simulink model "EdLuTSimulink"  (Simulink 8.1)
settings: Solver=ode3  StartTime=0.0  StopTime=1.  FixedStep=0.002  RelTol=1e-3
undefined symbols (not defined in the file or in its folder): frne
undefined symbols (not defined in the file): context, RRedKuKa, RRedKuKadet
libraries: simulink x1
(part 1 of 2)
settings Model: Creator=Sensopac  LastModifiedBy=jgarrido
settings DebuggingCC: StrictBusMsg=Warning
settings SFSimCC: SimParseCustomCode=off

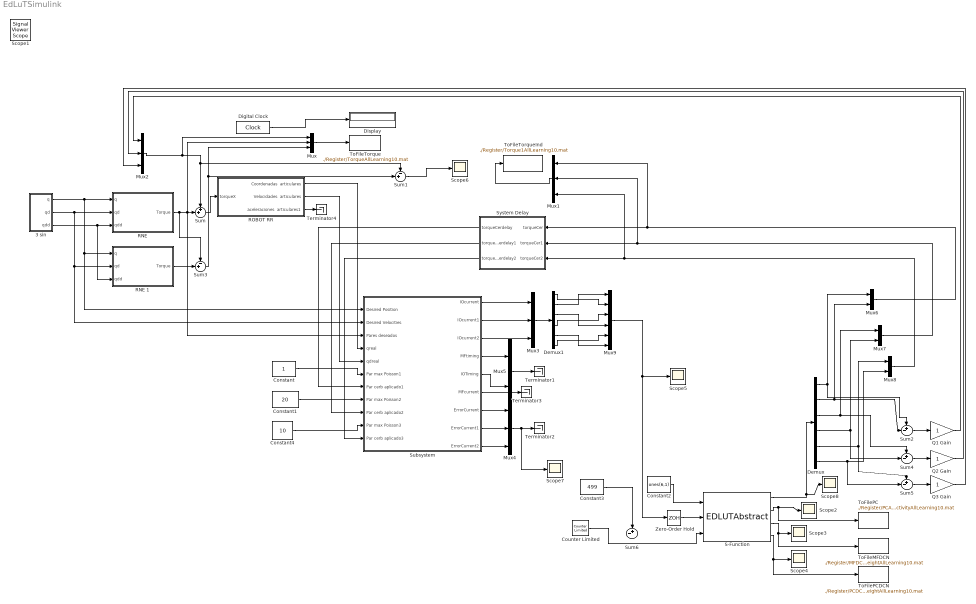
== system EdLuTSimulink ==
  3 sin : Subsystem
  Constant : Constant
  Constant1 : Constant  Value=20
  Constant2 : Constant  Value=ones(6,1)  OutDataTypeStr=double  SampleTime=0.002
  Constant3 : Constant  Value=499  OutDataTypeStr=double  SampleTime=0.002
  Constant4 : Constant  Value=10
  Counter Limited : simulink/Sources/Counter Limited  uplimit=499  tsamp=0.002
  Demux : Demux  Outputs=6
  Demux1 : Demux  Outputs=6
  Digital Clock : DigitalClock  SampleTime=0.002
  Display : Display
  Mux{,1..4} (5 alike) : Mux  Inputs=3
  Mux{5..8} (4 alike) : Mux  Inputs=2
  Mux9 : Mux  Inputs=6
  Q1 Gain : Gain
  Q2 Gain : Gain
  Q3 Gain : Gain
  "RNE " : Subsystem  mask{grav=[ 0 0 9.81], RRed=RRedKuKa}
      mask prompts: grav "Valor de gravedad( 0 0  -9.81)"; RRed "Robot"
      mask help:
      | Este bloque computa la dinamica inversa mediante la utilizacion del algoritmo
      | recursivo Newton Euler (computacionalmente mas eficiente que el metodo de
      | Lagrange-Euler)
      |
      | Se ha de introducir el valor de la gravedad con la que se ha de trabajar (direccion y modulo)
      mask Display:
      | port_label('output',1,'Torque')
      | port_label('input',1,'q')
      | port_label('input',2,'qd')
      | port_label('input',3,'qdd')
      | fprintf('RNE')
  RNE 1 : Subsystem  mask{grav=[ 0 0 9.81], RRed=RRedKuKadet}
      mask prompts: grav "Valor de gravedad( 0 0  -9.81)"; RRed "Robot"
      mask help:
      | Este bloque computa la dinamica inversa mediante la utilizacion del algoritmo
      | recursivo Newton Euler (computacionalmente mas eficiente que el metodo de
      | Lagrange-Euler)
      |
      | Se ha de introducir el valor de la gravedad con la que se ha de trabajar (direccion y modulo)
      mask Display:
      | port_label('output',1,'Torque')
      | port_label('input',1,'q')
      | port_label('input',2,'qd')
      | port_label('input',3,'qdd')
      | fprintf('RNE')
  ROBOT RR : Subsystem  mask{Ciniciales=[0.0  0.1*sin(pi/4)  0.1 0 0 0 0], Viniciales=[2*pi*0.1 2*pi*sin(pi/4)*0.1 0 0 0 0 0], RRed=RRedKuKadet}
      mask prompts: Ciniciales "Condiciones iniciales q"; Viniciales "Velocidades iniciales qd"; RRed "Robot"
      mask help: Modelado del brazo robotico mediante dinamica rigida
  S-Function : S-Function  FunctionName=EDLUTAbstract  Parameters=ParamFile NumberOfJoints NumberOfStates WeightFile WeightInitFile  EnableBusSupport=off  mask{ParamFile='Parametros.txt', NumberOfJoints=6, NumberOfStates=500, WeightFile='./Register/WeightsOnlyPC2_5.dat', WeightInitFile='./InitialWeights25.dat'}
      mask prompts: ParamFile "Learning Configuration File"; NumberOfJoints "Number Of Joints"; NumberOfStates "Number Of States"; WeightFile "Final Weight File"; WeightInitFile "Initial Weight File"
      mask Display:
      | port_label('input',1,'MFAct')
      | port_label('input',2,'Error')
      | port_label('input',3,'State')
      | port_label('output',1,'DCNAct')
      | port_label('output',2,'PCAct')
      | port_label('output',3,'MFWeight')
      | port_label('output',4,'PCWeight')
  Scope{2..8} (7 alike) : Scope
      Scope2 settings: TimeRange=10  YMin=0.3  YMax=1  SaveName=ScopeData3
      Scope3 settings: TimeRange=10  YMin=0  YMax=0.65  SaveName=ScopeData4
      Scope4 settings: TimeRange=20  YMin=6  YMax=80  SaveName=ScopeData5
      Scope5 settings: TimeRange=10  YMin=0  YMax=1
      Scope6 settings: TimeRange=20  YMin=-20  YMax=22.5  SaveName=ScopeData6
      Scope7 settings: TimeRange=10  YMin=-3  YMax=4  SaveName=ScopeData8
      Scope8 settings: TimeRange=10  YMin=0  YMax=17  SaveName=ScopeData9
  Subsystem : Subsystem
  Sum : Sum  Inputs=++|
  Sum1 : Sum  Inputs=-+|
  Sum2 : Sum  Inputs=+-|
  Sum3 : Sum  Inputs=-+|
  Sum4 : Sum  Inputs=+-|
  Sum5 : Sum  Inputs=+-|
  Sum6 : Sum  Inputs=+-|  OutDataTypeStr=uint16
  System Delay : Subsystem  mask{delta1=0}
      mask prompts: delta1 "Delay delta1"
  Terminator{1..4} (4 alike) : Terminator
  ToFileMFDCN : ToFile  Filename=./Register/MFDCNWeightAllLearning10.mat
  ToFilePC : ToFile  Filename=./Register/PCActivityAllLearning10.mat
  ToFilePCDCN : ToFile  Filename=./Register/PCDCNWeightAllLearning10.mat
  ToFileTorque : ToFile  Filename=./Register/TorqueAllLearning10.mat
  ToFileTorqueInd : ToFile  Filename=./Register/Torque1AllLearning10.mat
  Zero-Order Hold : ZeroOrderHold  SampleTime=0.002
  Scope1 : SignalViewerScope  IOType=viewer  RefreshTime=0.035000
  wires:
  3 sin/1(q) -> "RNE "/1(q), Subsystem/1(Desired Position), RNE 1/1(q)
  3 sin/2(qd) -> "RNE "/2(qd), Subsystem/2(Desired Velocities), RNE 1/2(qd)
  3 sin/3(qdd) -> "RNE "/3(qdd), RNE 1/3(qdd)
  "RNE "/1(Torque) -> Sum3/1, Sum/2, Mux/2, Subsystem/3(Pares deseados)
  ROBOT RR/1(Coordenadas  articulares) -> Subsystem/4(qreal)
  ROBOT RR/2(Velocidades  articulares) -> Subsystem/5(qdreal)
  Constant/1 -> Subsystem/6(Par max Poisson1)
  Constant1/1 -> Subsystem/8(Par max Poisson2)
  Constant4/1 -> Subsystem/10(Par max Poisson3)
  System Delay/1(torqueCerdelay) -> Subsystem/7(Par cerb aplicado1)
  System Delay/2(torqueCerdelay1) -> Subsystem/9(Par cerb aplicado2)
  System Delay/3(torqueCerdelay2) -> Subsystem/11(Par cerb aplicado3)
  Sum/1 -> ROBOT RR/1(torqueX)
  Subsystem/6(MFcurrent) -> Terminator3/1
  ROBOT RR/3(aceleraciones  articulares1) -> Terminator4/1
  Mux2/1 -> Sum/1, Sum1/1, Mux/1
  Mux/1 -> ToFileTorque/1
  Mux1/1 -> ToFileTorqueInd/1
  Constant2/1 -> S-Function/1
  S-Function/1 -> Demux/1, Scope8/1
  S-Function/2 -> Scope2/1, ToFilePC/1
  S-Function/3 -> Scope3/1, ToFileMFDCN/1
  S-Function/4 -> Scope4/1, ToFilePCDCN/1
  RNE 1/1(Torque) -> Sum3/2
  Sum3/1 -> Sum1/2, Mux/3
  Zero-Order Hold/1 -> S-Function/2
  Mux6/1 -> System Delay/1(torqueCer), Mux1/1
  Mux7/1 -> System Delay/2(torqueCer1), Mux1/2
  Mux8/1 -> System Delay/3(torqueCer2), Mux1/3
  Sum1/1 -> Scope6/1
  Demux/1 -> Sum2/1, Mux6/1
  Demux/3 -> Sum4/1, Mux7/1
  Demux/5 -> Sum5/1, Mux8/1
  Demux/6 -> Sum5/2, Mux8/2
  Demux/4 -> Sum4/2, Mux7/2
  Demux/2 -> Sum2/2, Mux6/2
  Mux5/1 -> Terminator1/1
  Mux4/1 -> Terminator2/1, Scope7/1
  Subsystem/5(IOTiming) -> Mux5/2
  Subsystem/4(MFtiming) -> Mux5/1
  Subsystem/7(ErrorCurrent) -> Mux4/1
  Subsystem/8(ErrorCurrent1) -> Mux4/2
  Subsystem/9(ErrorCurrent2) -> Mux4/3
  Mux3/1 -> Demux1/1
  Mux9/1 -> Zero-Order Hold/1, Scope5/1
  Demux1/2 -> Mux9/1
  Demux1/1 -> Mux9/2
  Demux1/3 -> Mux9/4
  Demux1/4 -> Mux9/3
  Demux1/5 -> Mux9/6
  Demux1/6 -> Mux9/5
  Subsystem/1(IOcurrent) -> Mux3/1
  Subsystem/2(IOcurrent1) -> Mux3/2
  Subsystem/3(IOcurrent2) -> Mux3/3
  Digital Clock/1 -> Display/1
  Constant3/1 -> Sum6/1
  Counter Limited/1 -> S-Function/3
  Sum2/1 -> Q1 Gain/1
  Q1 Gain/1 -> Mux2/1
  Sum4/1 -> Q2 Gain/1
  Q2 Gain/1 -> Mux2/2
  Sum5/1 -> Q3 Gain/1
  Q3 Gain/1 -> Mux2/3

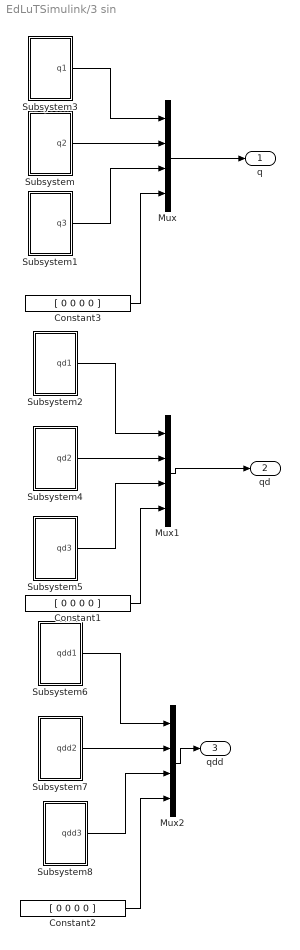
== system EdLuTSimulink/3 sin ==
  Constant1 : Constant  Value=[ 0 0 0 0 ]
  Constant2 : Constant  Value=[ 0 0 0 0 ]
  Constant3 : Constant  Value=[ 0 0 0 0 ]
  Mux : Mux
  Mux1 : Mux
  Mux2 : Mux
  Subsystem : Subsystem
  Subsystem1 : Subsystem
  Subsystem2 : Subsystem
  Subsystem3 : Subsystem
  Subsystem4 : Subsystem
  Subsystem5 : Subsystem
  Subsystem6 : Subsystem
  Subsystem7 : Subsystem
  Subsystem8 : Subsystem
  q : Outport
  qd : Outport  Port=2
  qdd : Outport  Port=3
  wires:
  Mux2/1 -> qdd/1
  Mux1/1 -> qd/1
  Mux/1 -> q/1
  Subsystem3/1(q1) -> Mux/1
  Subsystem/1(q2) -> Mux/2
  Subsystem1/1(q3) -> Mux/3
  Subsystem2/1(qd1) -> Mux1/1
  Subsystem4/1(qd2) -> Mux1/2
  Subsystem5/1(qd3) -> Mux1/3
  Subsystem6/1(qdd1) -> Mux2/1
  Subsystem7/1(qdd2) -> Mux2/2
  Subsystem8/1(qdd3) -> Mux2/3
  Constant3/1 -> Mux/4
  Constant1/1 -> Mux1/4
  Constant2/1 -> Mux2/4

== system EdLuTSimulink/RNE  ==
  q : Inport
  qd : Inport  Port=2
  qdd : Inport  Port=3
  Mux : Mux  Inputs=3
  S-Function : S-Function  FunctionName=Select  Parameters=RRed  EnableBusSupport=off
  S-Function1 : S-Function  FunctionName=Select  Parameters=RRed  EnableBusSupport=off
  S-Function2 : S-Function  FunctionName=Select  Parameters=RRed  EnableBusSupport=off
  rne : MATLABFcn  MATLABFcn=frne(RRed, u(1:RRed.n)', u(RRed.n+1:2*RRed.n)', u(2* RRed.n+1:3*RRed.n)',grav)  OutputDimensions=RRed.n
  Torque : Outport
  wires:
  qdd/1 -> S-Function2/1
  rne/1 -> Torque/1
  q/1 -> S-Function/1
  Mux/1 -> rne/1
  qd/1 -> S-Function1/1
  S-Function/1 -> Mux/1
  S-Function1/1 -> Mux/2
  S-Function2/1 -> Mux/3

== system EdLuTSimulink/RNE 1 ==
  q : Inport
  qd : Inport  Port=2
  qdd : Inport  Port=3
  Mux : Mux  Inputs=3
  S-Function : S-Function  FunctionName=Select  Parameters=RRed  EnableBusSupport=off
  S-Function1 : S-Function  FunctionName=Select  Parameters=RRed  EnableBusSupport=off
  S-Function2 : S-Function  FunctionName=Select  Parameters=RRed  EnableBusSupport=off
  rne : MATLABFcn  MATLABFcn=frne(RRed, u(1:RRed.n)', u(RRed.n+1:2*RRed.n)', u(2* RRed.n+1:3*RRed.n)',grav)  OutputDimensions=RRed.n
  Torque : Outport
  wires:
  qdd/1 -> S-Function2/1
  rne/1 -> Torque/1
  q/1 -> S-Function/1
  Mux/1 -> rne/1
  qd/1 -> S-Function1/1
  S-Function/1 -> Mux/1
  S-Function1/1 -> Mux/2
  S-Function2/1 -> Mux/3

== system EdLuTSimulink/ROBOT RR ==
  torqueX : Inport
  Constant : Constant  Value=Ciniciales
  Constant1 : Constant  Value=Viniciales
  Integrator : Integrator  ExternalReset=falling  InitialConditionSource=external
  Integrator1 : Integrator  ExternalReset=falling  InitialConditionSource=external
  Mux : Mux  Inputs=3
  Reset Contidions : Subsystem  mask{T=1}
      mask prompts: T "Period"
      mask Display: port_label ('output',1,'FallingReset')
  S-Function : S-Function  FunctionName=CINDIR  Parameters=RRed  EnableBusSupport=off
  S-Function1 : S-Function  FunctionName=Select  Parameters=RRed  EnableBusSupport=off
  S-Function2 : S-Function  FunctionName=Select  Parameters=RRed  EnableBusSupport=off
  Coordenadas  articulares : Outport
  Velocidades  articulares : Outport  Port=2
  aceleraciones  articulares1 : Outport  Port=3
  wires:
  torqueX/1 -> Mux/3
  Integrator/1 -> Integrator1/1, Mux/2, Velocidades  articulares/1  "qd"
  Mux/1 -> S-Function/1
  S-Function/1 -> Integrator/1, aceleraciones  articulares1/1  "qdd"
  Constant/1 -> S-Function1/1
  Integrator1/1 -> Mux/1, Coordenadas  articulares/1  "q"
  S-Function1/1 -> Integrator1/3
  S-Function2/1 -> Integrator/3
  Constant1/1 -> S-Function2/1
  Reset Contidions/1(Out1) -> Integrator1/2, Integrator/2

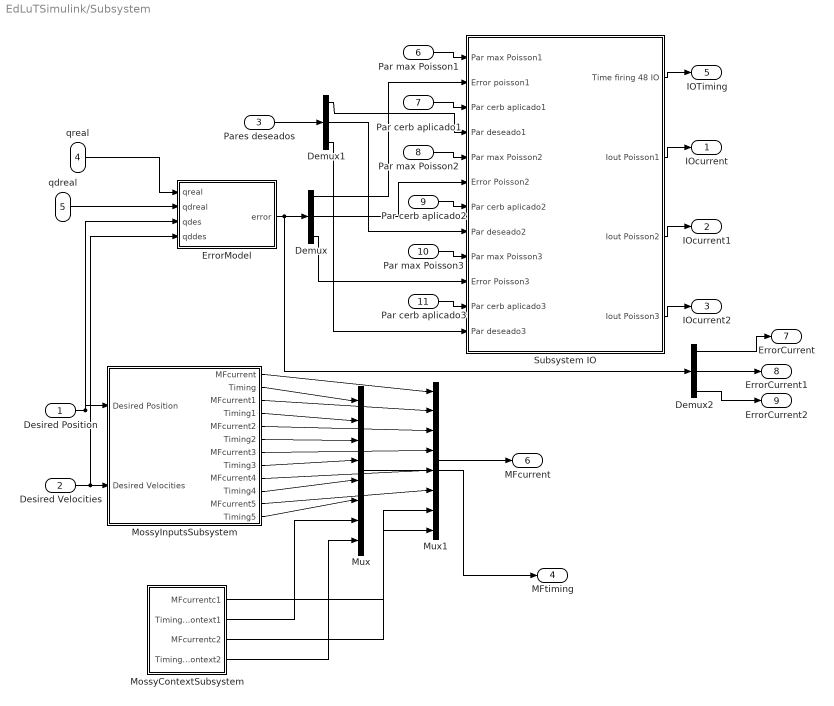
== system EdLuTSimulink/Subsystem ==
  Desired Position : Inport
  Desired Velocities : Inport  Port=2
  Pares deseados : Inport  Port=3
  qreal : Inport  Port=4
  qdreal : Inport  Port=5
  Par max Poisson1 : Inport  Port=6
  Par cerb aplicado1 : Inport  Port=7
  Par max Poisson2 : Inport  Port=8
  Par cerb aplicado2 : Inport  Port=9
  Par max Poisson3 : Inport  Port=10
  Par cerb aplicado3 : Inport  Port=11
  Demux : Demux  Outputs=3
  Demux1 : Demux  Outputs=3
  Demux2 : Demux  Outputs=3
  ErrorModel : Subsystem
  MossyContextSubsystem : Subsystem
  MossyInputsSubsystem : Subsystem
  Mux : Mux  Inputs=8
  Mux1 : Mux  Inputs=8
  Subsystem IO : Subsystem
  IOcurrent : Outport
  IOcurrent1 : Outport  Port=2
  IOcurrent2 : Outport  Port=3
  MFtiming : Outport  Port=4
  IOTiming : Outport  Port=5
  MFcurrent : Outport  Port=6
  ErrorCurrent : Outport  Port=7
  ErrorCurrent1 : Outport  Port=8
  ErrorCurrent2 : Outport  Port=9
  wires:
  Desired Position/1 -> MossyInputsSubsystem/1(Desired Position), ErrorModel/3(qdes)
  Desired Velocities/1 -> MossyInputsSubsystem/2(Desired Velocities), ErrorModel/4(qddes)
  Par max Poisson1/1 -> Subsystem IO/1(Par max Poisson1)
  Subsystem IO/1(Time firing 48 IO) -> IOTiming/1
  Demux/1 -> Subsystem IO/2(Error poisson1)
  Par cerb aplicado1/1 -> Subsystem IO/3(Par cerb aplicado1)
  Demux1/1 -> Subsystem IO/4(Par deseado1)
  Subsystem IO/2(Iout Poisson1) -> IOcurrent/1
  Par max Poisson2/1 -> Subsystem IO/5(Par max Poisson2)
  Demux/2 -> Subsystem IO/6(Error Poisson2)
  Par cerb aplicado2/1 -> Subsystem IO/7(Par cerb aplicado2)
  Subsystem IO/3(Iout Poisson2) -> IOcurrent1/1
  Par max Poisson3/1 -> Subsystem IO/9(Par max Poisson3)
  Demux/3 -> Subsystem IO/10(Error Poisson3)
  Par cerb aplicado3/1 -> Subsystem IO/11(Par cerb aplicado3)
  Subsystem IO/4(Iout Poisson3) -> IOcurrent2/1
  Demux1/3 -> Subsystem IO/12(Par deseado3)
  Pares deseados/1 -> Demux1/1
  ErrorModel/1(error) -> Demux/1, Demux2/1
  qreal/1 -> ErrorModel/1(qreal)
  qdreal/1 -> ErrorModel/2(qdreal)
  Demux1/2 -> Subsystem IO/8(Par deseado2)
  MossyInputsSubsystem/2(Timing) -> Mux/1
  MossyInputsSubsystem/4(Timing1) -> Mux/2
  MossyInputsSubsystem/6(Timing2) -> Mux/3
  MossyInputsSubsystem/8(Timing3) -> Mux/4
  MossyInputsSubsystem/10(Timing4) -> Mux/5
  MossyInputsSubsystem/12(Timing5) -> Mux/6
  MossyContextSubsystem/2(TimingContext1) -> Mux/7
  MossyContextSubsystem/4(TimingContext2) -> Mux/8
  Mux/1 -> MFtiming/1
  MossyInputsSubsystem/1(MFcurrent) -> Mux1/1
  MossyInputsSubsystem/3(MFcurrent1) -> Mux1/2
  MossyInputsSubsystem/5(MFcurrent2) -> Mux1/3
  MossyInputsSubsystem/7(MFcurrent3) -> Mux1/4
  MossyInputsSubsystem/9(MFcurrent4) -> Mux1/5
  MossyInputsSubsystem/11(MFcurrent5) -> Mux1/6
  MossyContextSubsystem/1(MFcurrentc1) -> Mux1/7
  MossyContextSubsystem/3(MFcurrentc2) -> Mux1/8
  Mux1/1 -> MFcurrent/1
  Demux2/1 -> ErrorCurrent/1
  Demux2/2 -> ErrorCurrent1/1
  Demux2/3 -> ErrorCurrent2/1

== system EdLuTSimulink/System Delay ==
  torqueCer : Inport
  torqueCer1 : Inport  Port=2
  torqueCer2 : Inport  Port=3
  Transport Delay1 : TransportDelay  DelayTime=delta1
  Transport Delay2 : TransportDelay  DelayTime=delta1
  Transport Delay3 : TransportDelay  DelayTime=delta1
  torqueCerdelay : Outport
  torqueCerdelay1 : Outport  Port=2
  torqueCerdelay2 : Outport  Port=3
  wires:
  torqueCer/1 -> Transport Delay1/1
  Transport Delay1/1 -> torqueCerdelay/1
  torqueCer1/1 -> Transport Delay2/1
  Transport Delay2/1 -> torqueCerdelay1/1
  torqueCer2/1 -> Transport Delay3/1
  Transport Delay3/1 -> torqueCerdelay2/1

== system EdLuTSimulink/3 sin/Subsystem ==
  Constant1 : Constant  Value=0.1
  Constant2 : Constant  Value=pi/4
  Constant3 : Constant  Value=2*pi
  Digital Clock : DigitalClock  SampleTime=0.002
  Product : Product  RndMeth=Zero
  Product2 : Product  RndMeth=Zero
  Sum : Sum  Inputs=|++
  Trigonometric Function : Trigonometry
  q2 : Outport
  wires:
  Sum/1 -> Trigonometric Function/1
  Constant2/1 -> Sum/1
  Product2/1 -> Sum/2
  Product/1 -> q2/1
  Trigonometric Function/1 -> Product/2
  Constant3/1 -> Product2/1
  Digital Clock/1 -> Product2/2
  Constant1/1 -> Product/1

== system EdLuTSimulink/3 sin/Subsystem1 ==
  Constant2 : Constant  Value=0.1
  Constant3 : Constant  Value=pi/2
  Constant4 : Constant  Value=2*pi
  Digital Clock : DigitalClock  SampleTime=0.002
  Product : Product  RndMeth=Zero
  Product2 : Product  RndMeth=Zero
  Sum : Sum  Inputs=|++
  Trigonometric Function : Trigonometry
  q3 : Outport
  wires:
  Sum/1 -> Trigonometric Function/1
  Constant3/1 -> Sum/1
  Product2/1 -> Sum/2
  Product/1 -> q3/1
  Trigonometric Function/1 -> Product/2
  Constant4/1 -> Product2/1
  Digital Clock/1 -> Product2/2
  Constant2/1 -> Product/1

== system EdLuTSimulink/3 sin/Subsystem2 ==
  Constant1 : Constant  Value=0.1*2*pi
  Constant3 : Constant  Value=2*pi
  Digital Clock : DigitalClock  SampleTime=0.002
  Product : Product  RndMeth=Zero
  Product2 : Product  RndMeth=Zero
  Trigonometric Function : Trigonometry  Operator=cos
  qd1 : Outport
  wires:
  Product/1 -> qd1/1
  Trigonometric Function/1 -> Product/2
  Constant3/1 -> Product2/1
  Product2/1 -> Trigonometric Function/1
  Digital Clock/1 -> Product2/2
  Constant1/1 -> Product/1

== system EdLuTSimulink/3 sin/Subsystem3 ==
  Constant1 : Constant  Value=0.1
  Constant3 : Constant  Value=2*pi
  Digital Clock : DigitalClock  SampleTime=0.002
  Product : Product  RndMeth=Zero
  Product2 : Product  RndMeth=Zero
  Trigonometric Function : Trigonometry
  q1 : Outport
  wires:
  Product/1 -> q1/1
  Trigonometric Function/1 -> Product/2
  Constant3/1 -> Product2/1
  Product2/1 -> Trigonometric Function/1
  Digital Clock/1 -> Product2/2
  Constant1/1 -> Product/1

== system EdLuTSimulink/3 sin/Subsystem4 ==
  Constant1 : Constant  Value=0.1*2*pi
  Constant2 : Constant  Value=pi/4
  Constant3 : Constant  Value=2*pi
  Digital Clock : DigitalClock  SampleTime=0.002
  Product : Product  RndMeth=Zero
  Product2 : Product  RndMeth=Zero
  Sum : Sum  Inputs=|++
  Trigonometric Function : Trigonometry  Operator=cos
  qd2 : Outport
  wires:
  Sum/1 -> Trigonometric Function/1
  Constant2/1 -> Sum/1
  Product2/1 -> Sum/2
  Product/1 -> qd2/1
  Trigonometric Function/1 -> Product/2
  Constant3/1 -> Product2/1
  Digital Clock/1 -> Product2/2
  Constant1/1 -> Product/1

== system EdLuTSimulink/3 sin/Subsystem5 ==
  Constant1 : Constant  Value=0.1*2*pi
  Constant3 : Constant  Value=pi/2
  Constant4 : Constant  Value=2*pi
  Digital Clock : DigitalClock  SampleTime=0.002
  Product : Product  RndMeth=Zero
  Product2 : Product  RndMeth=Zero
  Sum : Sum  Inputs=|++
  Trigonometric Function : Trigonometry  Operator=cos
  qd3 : Outport
  wires:
  Sum/1 -> Trigonometric Function/1
  Constant3/1 -> Sum/1
  Product2/1 -> Sum/2
  Product/1 -> qd3/1
  Trigonometric Function/1 -> Product/2
  Constant4/1 -> Product2/1
  Digital Clock/1 -> Product2/2
  Constant1/1 -> Product/1

== system EdLuTSimulink/3 sin/Subsystem6 ==
  Constant1 : Constant  Value=-0.1*4*pi^2
  Constant3 : Constant  Value=2*pi
  Digital Clock : DigitalClock  SampleTime=0.002
  Product : Product  RndMeth=Zero
  Product2 : Product  RndMeth=Zero
  Trigonometric Function : Trigonometry
  qdd1 : Outport
  wires:
  Product/1 -> qdd1/1
  Trigonometric Function/1 -> Product/2
  Constant3/1 -> Product2/1
  Product2/1 -> Trigonometric Function/1
  Digital Clock/1 -> Product2/2
  Constant1/1 -> Product/1

== system EdLuTSimulink/3 sin/Subsystem7 ==
  Constant1 : Constant  Value=-0.1*4*pi^2
  Constant2 : Constant  Value=pi/4
  Constant3 : Constant  Value=2*pi
  Digital Clock : DigitalClock  SampleTime=0.002
  Product : Product  RndMeth=Zero
  Product2 : Product  RndMeth=Zero
  Sum : Sum  Inputs=|++
  Trigonometric Function : Trigonometry
  qdd2 : Outport
  wires:
  Sum/1 -> Trigonometric Function/1
  Constant2/1 -> Sum/1
  Product2/1 -> Sum/2
  Product/1 -> qdd2/1
  Trigonometric Function/1 -> Product/2
  Constant3/1 -> Product2/1
  Digital Clock/1 -> Product2/2
  Constant1/1 -> Product/1

== system EdLuTSimulink/3 sin/Subsystem8 ==
  Constant1 : Constant  Value=-0.1*4*pi^2
  Constant3 : Constant  Value=pi/2
  Constant4 : Constant  Value=2*pi
  Digital Clock : DigitalClock  SampleTime=0.002
  Product : Product  RndMeth=Zero
  Product2 : Product  RndMeth=Zero
  Sum : Sum  Inputs=|++
  Trigonometric Function : Trigonometry
  qdd3 : Outport
  wires:
  Sum/1 -> Trigonometric Function/1
  Constant3/1 -> Sum/1
  Product2/1 -> Sum/2
  Product/1 -> qdd3/1
  Trigonometric Function/1 -> Product/2
  Constant4/1 -> Product2/1
  Digital Clock/1 -> Product2/2
  Constant1/1 -> Product/1

== system EdLuTSimulink/ROBOT RR/Reset Contidions ==
  Constant2 : Constant  Value=T
  Digital Clock : DigitalClock  SampleTime=0.002
  Math Function : Math  Operator=mod  OutputSignalType=real  SaturateOnIntegerOverflow=on
  Out1 : Outport
  wires:
  Digital Clock/1 -> Math Function/1
  Constant2/1 -> Math Function/2
  Math Function/1 -> Out1/1

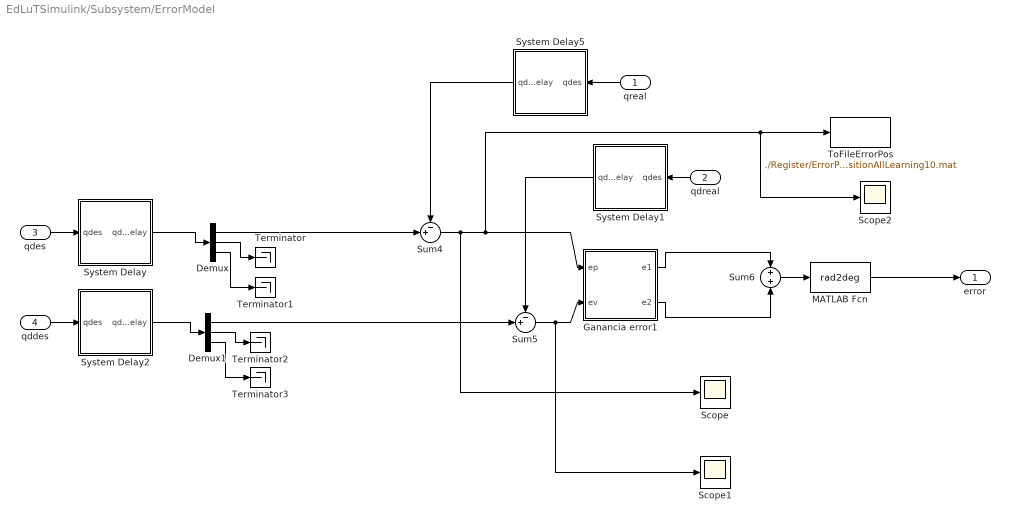
== system EdLuTSimulink/Subsystem/ErrorModel ==
  qreal : Inport
  qdreal : Inport  Port=2
  qdes : Inport  Port=3
  qddes : Inport  Port=4
  Demux : Demux  Outputs=3
  Demux1 : Demux  Outputs=3
  Ganancia error1 : Subsystem  mask{KP1=1, KP2=12, KP3=6, KV1=2, KV2=10, KV3=5}
      mask prompts: KP1 "Constante error de posición1"; KP2 "Constante error de posición2"; KP3 "Constante error de posición3"; KV1 "Constante error de velocidad1"; KV2 "Constante error de velocidad2"; KV3 "Constante error de velocidad3"
  MATLAB Fcn : MATLABFcn  MATLABFcn=rad2deg
  Scope : Scope
      settings: YMin=-0.02  YMax=0.15
  Scope1 : Scope
      settings: TimeRange=20  YMin=-0.05  YMax=0.375  SaveName=ScopeData2
  Scope2 : Scope
      settings: TimeRange=20  YMin=-0.005  YMax=0.0425  SaveName=ScopeData7
  Sum4 : Sum  Inputs=-+|
  Sum5 : Sum  Inputs=-+|
  Sum6 : Sum
  System Delay : Subsystem  mask{delta1=0, delta2=0, qinicial=[0.0  0.1*sin(pi/4)  0.1 0 0 0 0]}
      mask prompts: delta1 "Primer delay delta1"; delta2 "Segundo delay delta2"; qinicial "Posición inicial [q1 q2 q3 q4 q5 q6 q7]"
  System Delay1 : Subsystem  mask{delta1=0, delta2=0, qinicial=[2*pi*0.1 2*pi*sin(pi/4)*0.1 0]}
      mask prompts: delta1 "Primer delay delta1"; delta2 "Segundo delay delta2"; qinicial "Velocidad inicial [qd1 qd2 qd3]"
  System Delay2 : Subsystem  mask{delta1=0, delta2=0, qinicial=[2*pi*0.1 2*pi*sin(pi/4)*0.1 0 0 0 0 0]}
      mask prompts: delta1 "Primer delay delta1"; delta2 "Segundo delay delta2"; qinicial "Velocidad inicial [qd1 qd2 qd3 qd4 qd5 qd6 qd7]"
  System Delay5 : Subsystem  mask{delta1=0, delta2=0, qinicial=[0.0  0.1*sin(pi/4)  0.1]}
      mask prompts: delta1 "Primer delay delta1"; delta2 "Segundo delay delta2"; qinicial "Posición inicial [q1 q2 q3 ]"
  Terminator{,1..3} (4 alike) : Terminator
  ToFileErrorPos : ToFile  Filename=./Register/ErrorPositionAllLearning10.mat
  error : Outport
  wires:
  Sum4/1 -> Ganancia error1/1(ep), Scope2/1, ToFileErrorPos/1, Scope/1
  Sum5/1 -> Ganancia error1/2(ev), Scope1/1
  Ganancia error1/1(e1) -> Sum6/1
  Ganancia error1/2(e2) -> Sum6/2
  qreal/1 -> System Delay5/1(qdes)
  qdreal/1 -> System Delay1/1(qdes)
  qdes/1 -> System Delay/1(qdes)
  qddes/1 -> System Delay2/1(qdes)
  Sum6/1 -> MATLAB Fcn/1
  System Delay5/1(qdesdelay) -> Sum4/1
  System Delay1/1(qdesdelay) -> Sum5/1
  System Delay/1(qdesdelay) -> Demux/1
  System Delay2/1(qdesdelay) -> Demux1/1
  Demux/1 -> Sum4/2
  Demux1/1 -> Sum5/2
  Demux/2 -> Terminator/1
  Demux/3 -> Terminator1/1
  Demux1/2 -> Terminator2/1
  Demux1/3 -> Terminator3/1
  MATLAB Fcn/1 -> error/1

== system EdLuTSimulink/Subsystem/MossyContextSubsystem ==
  Contexto : Subsystem  mask{Variable_Contexto=context, Variable_Contexto1=context}
      mask prompts: Variable_Contexto "Variable de  contexto 1"; Variable_Contexto1 "Variable de contexto 2"
  Demux : Demux  Outputs=2
  Mossy1 : Subsystem  mask{R=5, Taum=0.02, Um0=0, Uth=1, Ureset=0, Trefrac=0, NumMFs=4}
      mask prompts: R "Valor R"; Um0 "Valor inicial de Um"; Uth "Tensión Th"; Ureset "Tensión Reset"; Trefrac "Tiempo Refractario"; NumMFs "Numero de MFs"
      mask Display:
      | port_label('input',1,'MFs inputs')
      | port_label('output',1,'MFs potential')
      | port_label('output',2,'Firing MFs')
  Mossy7 : Subsystem  mask{R=5, Taum=0.02, Um0=0, Uth=1, Ureset=0, Trefrac=0, NumMFs=4}
      mask prompts: R "Valor R"; Um0 "Valor inicial de Um"; Uth "Tensión Th"; Ureset "Tensión Reset"; Trefrac "Tiempo Refractario"; NumMFs "Numero de MFs"
      mask Display:
      | port_label('input',1,'MFs inputs')
      | port_label('output',1,'MFs potential')
      | port_label('output',2,'Firing MFs')
  Mux : Mux
  Mux1 : Mux
  RBFdesired2 : S-Function  FunctionName=fRBFdesiredcontex1optimal  Parameters=PasoGradocontext1,numRBFs,sigmacontext1,limitinfcontext1,limitsupcontext1,maxforcecontext1  EnableBusSupport=off  mask{PasoGradocontext1=0.1, numRBFs=2, sigmacontext1=3, limitinfcontext1=0, limitsupcontext1=10, maxforcecontext1=10}
      mask prompts: PasoGradocontext1 "Paso de Grado"; numRBFs "Número de RBFs"; sigmacontext1 "sigma"; limitinfcontext1 "limite inferior"; limitsupcontext1 "limit superior"; maxforcecontext1 "Fuerza máxima aplicable"
      mask help: Se ha de tener en consideración cual es la magnitud del error con el que se va a trabajar, de manera que, los límites inferior y superior así como el paso de muestreo estén en consonancia con dicha magnitud
  Terminator : Terminator
  MFcurrentc1 : Outport
  TimingContext1 : Outport  Port=2
  MFcurrentc2 : Outport  Port=3
  TimingContext2 : Outport  Port=4
  wires:
  Contexto/1(Context Variable1) -> RBFdesired2/1
  Contexto/2(Context Variable 2) -> Terminator/1
  Demux/1 -> Mux/1, Mux/2, Mux/3, Mux/4
  Demux/2 -> Mux1/1, Mux1/2, Mux1/3, Mux1/4
  RBFdesired2/1 -> Demux/1
  Mossy1/1(Out1) -> MFcurrentc1/1
  Mossy1/2(Out2) -> TimingContext1/1
  Mossy7/1(Out1) -> MFcurrentc2/1
  Mossy7/2(Out2) -> TimingContext2/1
  Mux/1 -> Mossy1/1(In1)
  Mux1/1 -> Mossy7/1(In1)

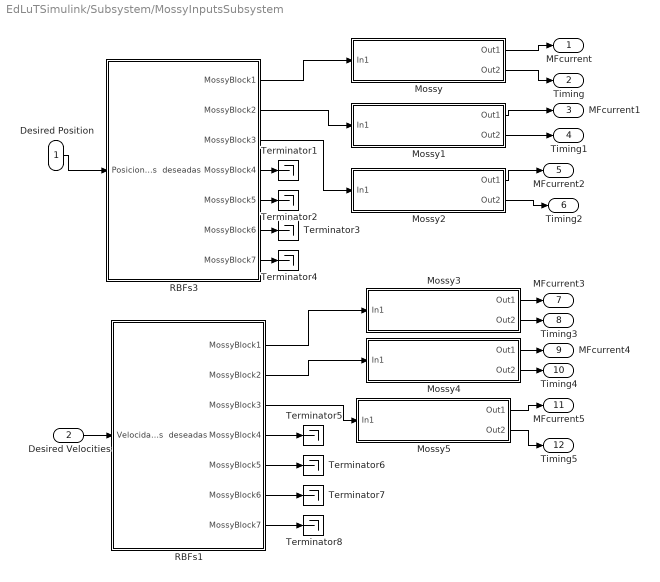
== system EdLuTSimulink/Subsystem/MossyInputsSubsystem ==
  Desired Position : Inport
  Desired Velocities : Inport  Port=2
  Mossy : Subsystem  mask{R=5, Taum=0.02, Um0=0, Uth=1, Ureset=0, Trefrac=0, NumMFs=20}
      mask prompts: R "Valor R"; Um0 "Valor inicial de Um"; Uth "Tensión Th"; Ureset "Tensión Reset"; Trefrac "Tiempo Refractario"; NumMFs "Numero de MFs"
      mask Display:
      | port_label('input',1,'MFs inputs')
      | port_label('output',1,'MFs potential')
      | port_label('output',2,'Firing MFs')
  Mossy1 : Subsystem  mask{R=5, Taum=0.02, Um0=0, Uth=1, Ureset=0, Trefrac=0, NumMFs=20}
      mask prompts: R "Valor R"; Um0 "Valor inicial de Um"; Uth "Tensión Th"; Ureset "Tensión Reset"; Trefrac "Tiempo Refractario"; NumMFs "Numero de MFs"
      mask Display:
      | port_label('input',1,'MFs inputs')
      | port_label('output',1,'MFs potential')
      | port_label('output',2,'Firing MFs')
  Mossy2 : Subsystem  mask{R=5, Taum=0.02, Um0=0, Uth=1, Ureset=0, Trefrac=0, NumMFs=20}
      mask prompts: R "Valor R"; Um0 "Valor inicial de Um"; Uth "Tensión Th"; Ureset "Tensión Reset"; Trefrac "Tiempo Refractario"; NumMFs "Numero de MFs"
      mask Display:
      | port_label('input',1,'MFs inputs')
      | port_label('output',1,'MFs potential')
      | port_label('output',2,'Firing MFs')
  Mossy3 : Subsystem  mask{R=5, Taum=0.02, Um0=0, Uth=1, Ureset=0, Trefrac=0, NumMFs=20}
      mask prompts: R "Valor R"; Um0 "Valor inicial de Um"; Uth "Tensión Th"; Ureset "Tensión Reset"; Trefrac "Tiempo Refractario"; NumMFs "Numero de MFs"
      mask Display:
      | port_label('input',1,'MFs inputs')
      | port_label('output',1,'MFs potential')
      | port_label('output',2,'Firing MFs')
  Mossy4 : Subsystem  mask{R=5, Taum=0.02, Um0=0, Uth=1, Ureset=0, Trefrac=0, NumMFs=20}
      mask prompts: R "Valor R"; Um0 "Valor inicial de Um"; Uth "Tensión Th"; Ureset "Tensión Reset"; Trefrac "Tiempo Refractario"; NumMFs "Numero de MFs"
      mask Display:
      | port_label('input',1,'MFs inputs')
      | port_label('output',1,'MFs potential')
      | port_label('output',2,'Firing MFs')
  Mossy5 : Subsystem  mask{R=5, Taum=0.02, Um0=0, Uth=1, Ureset=0, Trefrac=0, NumMFs=20}
      mask prompts: R "Valor R"; Um0 "Valor inicial de Um"; Uth "Tensión Th"; Ureset "Tensión Reset"; Trefrac "Tiempo Refractario"; NumMFs "Numero de MFs"
      mask Display:
      | port_label('input',1,'MFs inputs')
      | port_label('output',1,'MFs potential')
      | port_label('output',2,'Firing MFs')
  RBFs1 : Subsystem
  RBFs3 : Subsystem
  Terminator{1..8} (8 alike) : Terminator
  MFcurrent : Outport
  Timing : Outport  Port=2
  MFcurrent1 : Outport  Port=3
  Timing1 : Outport  Port=4
  MFcurrent2 : Outport  Port=5
  Timing2 : Outport  Port=6
  MFcurrent3 : Outport  Port=7
  Timing3 : Outport  Port=8
  MFcurrent4 : Outport  Port=9
  Timing4 : Outport  Port=10
  MFcurrent5 : Outport  Port=11
  Timing5 : Outport  Port=12
  wires:
  RBFs3/1(MossyBlock1) -> Mossy/1(In1)
  RBFs3/2(MossyBlock2) -> Mossy1/1(In1)
  RBFs3/3(MossyBlock3) -> Mossy2/1(In1)
  RBFs3/4(MossyBlock4) -> Terminator1/1
  RBFs3/5(MossyBlock5) -> Terminator2/1
  RBFs3/6(MossyBlock6) -> Terminator3/1
  RBFs3/7(MossyBlock7) -> Terminator4/1
  RBFs1/1(MossyBlock1) -> Mossy3/1(In1)
  RBFs1/2(MossyBlock2) -> Mossy4/1(In1)
  RBFs1/3(MossyBlock3) -> Mossy5/1(In1)
  RBFs1/4(MossyBlock4) -> Terminator5/1
  RBFs1/5(MossyBlock5) -> Terminator6/1
  RBFs1/6(MossyBlock6) -> Terminator7/1
  RBFs1/7(MossyBlock7) -> Terminator8/1
  Desired Position/1 -> RBFs3/1(Posiciones  deseadas)
  Desired Velocities/1 -> RBFs1/1(Velocidades  deseadas)
  Mossy/1(Out1) -> MFcurrent/1
  Mossy/2(Out2) -> Timing/1
  Mossy1/1(Out1) -> MFcurrent1/1
  Mossy1/2(Out2) -> Timing1/1
  Mossy2/1(Out1) -> MFcurrent2/1
  Mossy2/2(Out2) -> Timing2/1
  Mossy3/1(Out1) -> MFcurrent3/1
  Mossy3/2(Out2) -> Timing3/1
  Mossy4/1(Out1) -> MFcurrent4/1
  Mossy4/2(Out2) -> Timing4/1
  Mossy5/1(Out1) -> MFcurrent5/1
  Mossy5/2(Out2) -> Timing5/1

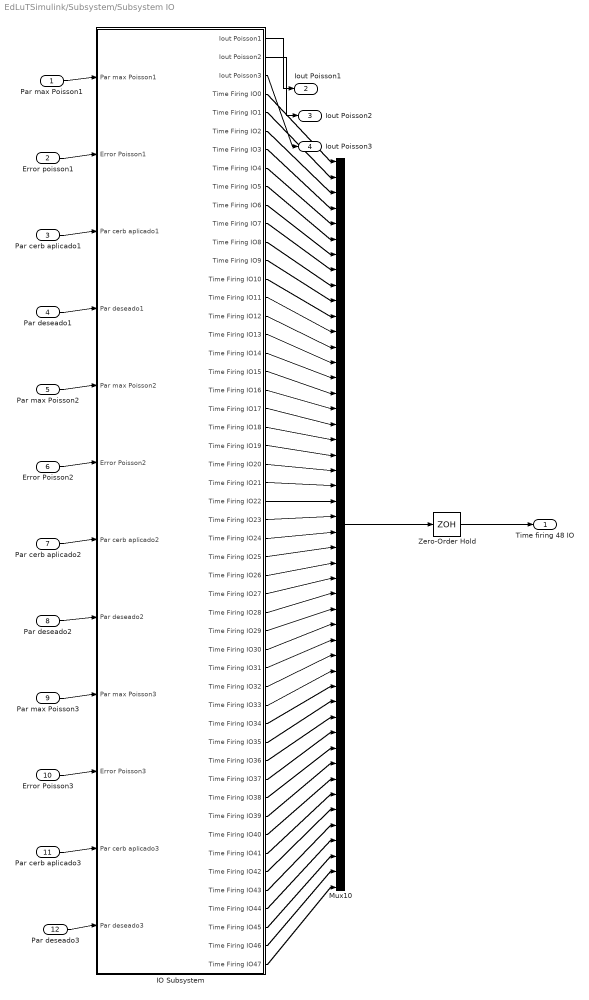
== system EdLuTSimulink/Subsystem/Subsystem IO ==
  Par max Poisson1 : Inport
  Error poisson1 : Inport  Port=2
  Par cerb aplicado1 : Inport  Port=3
  Par deseado1 : Inport  Port=4
  Par max Poisson2 : Inport  Port=5
  Error Poisson2 : Inport  Port=6
  Par cerb aplicado2 : Inport  Port=7
  Par deseado2 : Inport  Port=8
  Par max Poisson3 : Inport  Port=9
  Error Poisson3 : Inport  Port=10
  Par cerb aplicado3 : Inport  Port=11
  Par deseado3 : Inport  Port=12
  "IO Subsystem " : Subsystem
  Mux10 : Mux  Inputs=48
  Zero-Order Hold : ZeroOrderHold  SampleTime=0.002
  Time firing 48 IO : Outport
  Iout Poisson1 : Outport  Port=2
  Iout Poisson2 : Outport  Port=3
  Iout Poisson3 : Outport  Port=4
  wires:
  Par max Poisson1/1 -> "IO Subsystem "/1(Par max Poisson1)
  Error poisson1/1 -> "IO Subsystem "/2(Error Poisson1)
  Par deseado1/1 -> "IO Subsystem "/4(Par deseado1)
  Par max Poisson2/1 -> "IO Subsystem "/5(Par max Poisson2)
  Error Poisson2/1 -> "IO Subsystem "/6(Error Poisson2)
  Par deseado2/1 -> "IO Subsystem "/8(Par deseado2)
  Par cerb aplicado2/1 -> "IO Subsystem "/7(Par cerb aplicado2)
  Par cerb aplicado1/1 -> "IO Subsystem "/3(Par cerb aplicado1)
  "IO Subsystem "/1(Iout Poisson1) -> Iout Poisson1/1
  "IO Subsystem "/2(Iout Poisson2) -> Iout Poisson2/1
  "IO Subsystem "/3(Iout Poisson3) -> Iout Poisson3/1
  Par max Poisson3/1 -> "IO Subsystem "/9(Par max Poisson3)
  Error Poisson3/1 -> "IO Subsystem "/10(Error Poisson3)
  Par cerb aplicado3/1 -> "IO Subsystem "/11(Par cerb aplicado3)
  Par deseado3/1 -> "IO Subsystem "/12(Par deseado3)
  "IO Subsystem "/51(Time Firing IO47) -> Mux10/48
  "IO Subsystem "/4(Time Firing IO0) -> Mux10/1
  "IO Subsystem "/5(Time Firing IO1) -> Mux10/2
  "IO Subsystem "/6(Time Firing IO2) -> Mux10/3
  "IO Subsystem "/7(Time Firing IO3) -> Mux10/4
  "IO Subsystem "/8(Time Firing IO4) -> Mux10/5
  "IO Subsystem "/9(Time Firing IO5) -> Mux10/6
  "IO Subsystem "/10(Time Firing IO6) -> Mux10/7
  "IO Subsystem "/11(Time Firing IO7) -> Mux10/8
  "IO Subsystem "/12(Time Firing IO8) -> Mux10/9
  "IO Subsystem "/13(Time Firing IO9) -> Mux10/10
  "IO Subsystem "/14(Time Firing IO10) -> Mux10/11
  "IO Subsystem "/15(Time Firing IO11) -> Mux10/12
  "IO Subsystem "/16(Time Firing IO12) -> Mux10/13
  "IO Subsystem "/17(Time Firing IO13) -> Mux10/14
  "IO Subsystem "/18(Time Firing IO14) -> Mux10/15
  "IO Subsystem "/19(Time Firing IO15) -> Mux10/16
  "IO Subsystem "/20(Time Firing IO16) -> Mux10/17
  "IO Subsystem "/21(Time Firing IO17) -> Mux10/18
  "IO Subsystem "/22(Time Firing IO18) -> Mux10/19
  "IO Subsystem "/23(Time Firing IO19) -> Mux10/20
  "IO Subsystem "/24(Time Firing IO20) -> Mux10/21
  "IO Subsystem "/50(Time Firing IO46) -> Mux10/47
  "IO Subsystem "/49(Time Firing IO45) -> Mux10/46
  "IO Subsystem "/48(Time Firing IO44) -> Mux10/45
  "IO Subsystem "/47(Time Firing IO43) -> Mux10/44
  "IO Subsystem "/46(Time Firing IO42) -> Mux10/43
  "IO Subsystem "/45(Time Firing IO41) -> Mux10/42
  "IO Subsystem "/44(Time Firing IO40) -> Mux10/41
  "IO Subsystem "/43(Time Firing IO39) -> Mux10/40
  "IO Subsystem "/42(Time Firing IO38) -> Mux10/39
  "IO Subsystem "/41(Time Firing IO37) -> Mux10/38
  "IO Subsystem "/40(Time Firing IO36) -> Mux10/37
  "IO Subsystem "/39(Time Firing IO35) -> Mux10/36
  "IO Subsystem "/38(Time Firing IO34) -> Mux10/35
  "IO Subsystem "/37(Time Firing IO33) -> Mux10/34
  "IO Subsystem "/36(Time Firing IO32) -> Mux10/33
  "IO Subsystem "/35(Time Firing IO31) -> Mux10/32
  "IO Subsystem "/34(Time Firing IO30) -> Mux10/31
  "IO Subsystem "/32(Time Firing IO28) -> Mux10/29
  "IO Subsystem "/33(Time Firing IO29) -> Mux10/30
  "IO Subsystem "/31(Time Firing IO27) -> Mux10/28
  "IO Subsystem "/30(Time Firing IO26) -> Mux10/27
  "IO Subsystem "/29(Time Firing IO25) -> Mux10/26
  "IO Subsystem "/28(Time Firing IO24) -> Mux10/25
  "IO Subsystem "/27(Time Firing IO23) -> Mux10/24
  "IO Subsystem "/26(Time Firing IO22) -> Mux10/23
  "IO Subsystem "/25(Time Firing IO21) -> Mux10/22
  Mux10/1 -> Zero-Order Hold/1
  Zero-Order Hold/1 -> Time firing 48 IO/1

== system EdLuTSimulink/Subsystem/ErrorModel/Ganancia error1 ==
  ep : Inport
  ev : Inport  Port=2
  Gain : Gain  Gain=[KP1 0 0;0 KP2 0;0 0 KP3]  Multiplication=Matrix(K*u)
  Gain1 : Gain  Gain=[KV1 0 0;0 KV2 0; 0 0 KV3]  Multiplication=Matrix(K*u)
  e1 : Outport
  e2 : Outport  Port=2
  wires:
  ep/1 -> Gain/1
  ev/1 -> Gain1/1
  Gain/1 -> e1/1
  Gain1/1 -> e2/1

== system EdLuTSimulink/Subsystem/ErrorModel/System Delay ==
  qdes : Inport
  Transport Delay : TransportDelay  DelayTime=delta1  InitialOutput=qinicial
  Transport Delay1 : TransportDelay  DelayTime=delta2  InitialOutput=qinicial
  qdesdelay : Outport
  wires:
  Transport Delay/1 -> Transport Delay1/1
  qdes/1 -> Transport Delay/1
  Transport Delay1/1 -> qdesdelay/1

== system EdLuTSimulink/Subsystem/ErrorModel/System Delay1 ==
  qdes : Inport
  Transport Delay : TransportDelay  DelayTime=delta1  InitialOutput=qinicial
  Transport Delay1 : TransportDelay  DelayTime=delta2  InitialOutput=qinicial
  qdesdelay : Outport
  wires:
  Transport Delay/1 -> Transport Delay1/1
  qdes/1 -> Transport Delay/1
  Transport Delay1/1 -> qdesdelay/1

== system EdLuTSimulink/Subsystem/ErrorModel/System Delay2 ==
  qdes : Inport
  Transport Delay : TransportDelay  DelayTime=delta1  InitialOutput=qinicial
  Transport Delay1 : TransportDelay  DelayTime=delta2  InitialOutput=qinicial
  qdesdelay : Outport
  wires:
  Transport Delay/1 -> Transport Delay1/1
  qdes/1 -> Transport Delay/1
  Transport Delay1/1 -> qdesdelay/1

== system EdLuTSimulink/Subsystem/ErrorModel/System Delay5 ==
  qdes : Inport
  Transport Delay : TransportDelay  DelayTime=delta1  InitialOutput=qinicial
  Transport Delay1 : TransportDelay  DelayTime=delta2  InitialOutput=qinicial
  qdesdelay : Outport
  wires:
  Transport Delay/1 -> Transport Delay1/1
  qdes/1 -> Transport Delay/1
  Transport Delay1/1 -> qdesdelay/1

== system EdLuTSimulink/Subsystem/MossyContextSubsystem/Contexto ==
  Constant : Constant  Value=Variable_Contexto
  Constant1 : Constant  Value=Variable_Contexto1
  Context Variable1 : Outport
  Context Variable 2 : Outport  Port=2
  wires:
  Constant/1 -> Context Variable1/1
  Constant1/1 -> Context Variable 2/1

== system EdLuTSimulink/Subsystem/MossyContextSubsystem/Mossy1 ==
  In1 : Inport
  Mossy : Subsystem  mask{R=R, Taum=Taum, Um0=Um0, Uth=Uth, Ureset=Ureset, Trefract=Trefrac, NumMFs=NumMFs}
      mask prompts: R "Valor R"; Um0 "Valor inicial de Um"; Uth "Tensión Th"; Ureset "Tensión Reset"; Trefract "Tiempo refractario"; NumMFs "CantidadMFs"
  Out1 : Outport
  Out2 : Outport  Port=2
  wires:
  In1/1 -> Mossy/1(I(t))
  Mossy/1(Um) -> Out1/1
  Mossy/2(mossyfire) -> Out2/1

== system EdLuTSimulink/Subsystem/MossyContextSubsystem/Mossy7 ==
  In1 : Inport
  Mossy : Subsystem  mask{R=R, Taum=Taum, Um0=Um0, Uth=Uth, Ureset=Ureset, Trefract=Trefrac, NumMFs=NumMFs}
      mask prompts: R "Valor R"; Um0 "Valor inicial de Um"; Uth "Tensión Th"; Ureset "Tensión Reset"; Trefract "Tiempo refractario"; NumMFs "CantidadMFs"
  Out1 : Outport
  Out2 : Outport  Port=2
  wires:
  In1/1 -> Mossy/1(I(t))
  Mossy/1(Um) -> Out1/1
  Mossy/2(mossyfire) -> Out2/1

== system EdLuTSimulink/Subsystem/MossyInputsSubsystem/Mossy ==
  In1 : Inport
  Mossy : Subsystem  mask{R=R, Taum=Taum, Um0=Um0, Uth=Uth, Ureset=Ureset, Trefract=Trefrac, NumMFs=NumMFs}
      mask prompts: R "Valor R"; Um0 "Valor inicial de Um"; Uth "Tensión Th"; Ureset "Tensión Reset"; Trefract "Tiempo refractario"; NumMFs "CantidadMFs"
  Out1 : Outport
  Out2 : Outport  Port=2
  wires:
  In1/1 -> Mossy/1(I(t))
  Mossy/1(Um) -> Out1/1
  Mossy/2(mossyfire) -> Out2/1

== system EdLuTSimulink/Subsystem/MossyInputsSubsystem/Mossy1 ==
  In1 : Inport
  Mossy : Subsystem  mask{R=R, Taum=Taum, Um0=Um0, Uth=Uth, Ureset=Ureset, Trefract=Trefrac, NumMFs=NumMFs}
      mask prompts: R "Valor R"; Um0 "Valor inicial de Um"; Uth "Tensión Th"; Ureset "Tensión Reset"; Trefract "Tiempo refractario"; NumMFs "CantidadMFs"
  Out1 : Outport
  Out2 : Outport  Port=2
  wires:
  In1/1 -> Mossy/1(I(t))
  Mossy/1(Um) -> Out1/1
  Mossy/2(mossyfire) -> Out2/1

== system EdLuTSimulink/Subsystem/MossyInputsSubsystem/Mossy2 ==
  In1 : Inport
  Mossy : Subsystem  mask{R=R, Taum=Taum, Um0=Um0, Uth=Uth, Ureset=Ureset, Trefract=Trefrac, NumMFs=NumMFs}
      mask prompts: R "Valor R"; Um0 "Valor inicial de Um"; Uth "Tensión Th"; Ureset "Tensión Reset"; Trefract "Tiempo refractario"; NumMFs "CantidadMFs"
  Out1 : Outport
  Out2 : Outport  Port=2
  wires:
  In1/1 -> Mossy/1(I(t))
  Mossy/1(Um) -> Out1/1
  Mossy/2(mossyfire) -> Out2/1

== system EdLuTSimulink/Subsystem/MossyInputsSubsystem/Mossy3 ==
  In1 : Inport
  Mossy : Subsystem  mask{R=R, Taum=Taum, Um0=Um0, Uth=Uth, Ureset=Ureset, Trefract=Trefrac, NumMFs=NumMFs}
      mask prompts: R "Valor R"; Um0 "Valor inicial de Um"; Uth "Tensión Th"; Ureset "Tensión Reset"; Trefract "Tiempo refractario"; NumMFs "CantidadMFs"
  Out1 : Outport
  Out2 : Outport  Port=2
  wires:
  In1/1 -> Mossy/1(I(t))
  Mossy/1(Um) -> Out1/1
  Mossy/2(mossyfire) -> Out2/1

== system EdLuTSimulink/Subsystem/MossyInputsSubsystem/Mossy4 ==
  In1 : Inport
  Mossy : Subsystem  mask{R=R, Taum=Taum, Um0=Um0, Uth=Uth, Ureset=Ureset, Trefract=Trefrac, NumMFs=NumMFs}
      mask prompts: R "Valor R"; Um0 "Valor inicial de Um"; Uth "Tensión Th"; Ureset "Tensión Reset"; Trefract "Tiempo refractario"; NumMFs "CantidadMFs"
  Out1 : Outport
  Out2 : Outport  Port=2
  wires:
  In1/1 -> Mossy/1(I(t))
  Mossy/1(Um) -> Out1/1
  Mossy/2(mossyfire) -> Out2/1

== system EdLuTSimulink/Subsystem/MossyInputsSubsystem/Mossy5 ==
  In1 : Inport
  Mossy : Subsystem  mask{R=R, Taum=Taum, Um0=Um0, Uth=Uth, Ureset=Ureset, Trefract=Trefrac, NumMFs=NumMFs}
      mask prompts: R "Valor R"; Um0 "Valor inicial de Um"; Uth "Tensión Th"; Ureset "Tensión Reset"; Trefract "Tiempo refractario"; NumMFs "CantidadMFs"
  Out1 : Outport
  Out2 : Outport  Port=2
  wires:
  In1/1 -> Mossy/1(I(t))
  Mossy/1(Um) -> Out1/1
  Mossy/2(mossyfire) -> Out2/1

== system EdLuTSimulink/Subsystem/MossyInputsSubsystem/RBFs1 ==
  Velocidades  deseadas : Inport
  Demux : Demux  Outputs=7
  MATLAB Fcn7 : MATLABFcn  MATLABFcn=rad2deg(u)
  S1 : S-Function  FunctionName=fRBFgausspeed1optimal  Parameters=PasoGrado1,numRBFs,sigma1,limitinf1,limitsup1,numfig,ver  EnableBusSupport=off  mask{PasoGrado1=0.1, numRBFs=20, sigma1=(36-(-36))/(1.75*20), limitinf1=-36, limitsup1=36, numfig=1, ver=0}
      mask prompts: PasoGrado1 "Tamaño de paso de grado"; numRBFs "Número de RBFs"; sigma1 "Sigma"; limitinf1 "Límite inferior"; limitsup1 "Límite superior"; numfig "Numero de figura"; ver "Visualización de gráficas VER=1"
  S2 : S-Function  FunctionName=fRBFgausspeed1optimal  Parameters=PasoGrado2,numRBFs,sigma2,limitinf2,limitsup2,numfig,ver  EnableBusSupport=off  mask{PasoGrado2=0.1, numRBFs=20, sigma2=(36-(-36))/(1.75*20), limitinf2=-36, limitsup2=36, numfig=2, ver=0}
      mask prompts: PasoGrado2 "Tamaño de paso de grado"; numRBFs "Número de RBFs"; sigma2 "Sigma"; limitinf2 "Límite inferior"; limitsup2 "Límite superior"; numfig "Numero de figura"; ver "Visualización de gráficas VER=1"
  S3 : S-Function  FunctionName=fRBFgausspeed1optimal  Parameters=PasoGrado3,numRBFs,sigma3,limitinf3,limitsup3,numfig,ver  EnableBusSupport=off  mask{PasoGrado3=0.1, numRBFs=20, sigma3=(36-(-36))/(1.75*20), limitinf3=-36, limitsup3=36, numfig=2, ver=0}
      mask prompts: PasoGrado3 "Tamaño de paso de grado"; numRBFs "Número de RBFs"; sigma3 "Sigma"; limitinf3 "Límite inferior"; limitsup3 "Límite superior"; numfig "Numero de figura"; ver "Visualización de gráficas VER=1"
  MossyBlock1 : Outport
  MossyBlock2 : Outport  Port=2
  MossyBlock3 : Outport  Port=3
  MossyBlock4 : Outport  Port=4
  MossyBlock5 : Outport  Port=5
  MossyBlock6 : Outport  Port=6
  MossyBlock7 : Outport  Port=7
  wires:
  Demux/1 -> S1/1
  Demux/2 -> S2/1
  S1/1 -> MossyBlock1/1
  S2/1 -> MossyBlock2/1
  Demux/3 -> S3/1
  Demux/4 -> MossyBlock4/1
  Demux/5 -> MossyBlock5/1
  Demux/6 -> MossyBlock6/1
  Demux/7 -> MossyBlock7/1
  MATLAB Fcn7/1 -> Demux/1
  Velocidades  deseadas/1 -> MATLAB Fcn7/1
  S3/1 -> MossyBlock3/1

== system EdLuTSimulink/Subsystem/MossyInputsSubsystem/RBFs3 ==
  Posiciones  deseadas : Inport
  Demux : Demux  Outputs=7
  MATLAB Fcn7 : MATLABFcn  MATLABFcn=rad2deg(u)
  S1 : S-Function  FunctionName=fRBFgauss1optimal  Parameters=PasoGrado1,numRBFs,sigma1,limitinf1,limitsup1,numfig,ver  EnableBusSupport=off  mask{PasoGrado1=0.05, numRBFs=20, sigma1=(6-(-6))/(1.75*20), limitinf1=-6, limitsup1=6, numfig=1, ver=0}
      mask prompts: PasoGrado1 "Tamaño de paso de grado"; numRBFs "Número de RBFs"; sigma1 "Sigma"; limitinf1 "Límite inferior"; limitsup1 "Límite superior"; numfig "Numero de figura"; ver "Visualización de gráficas VER=1"
  S2 : S-Function  FunctionName=fRBFgauss1optimal  Parameters=PasoGrado2,numRBFs,sigma2,limitinf2,limitsup2,numfig,ver  EnableBusSupport=off  mask{PasoGrado2=0.05, numRBFs=20, sigma2=(6-(-6))/(1.75*20), limitinf2=-6, limitsup2=6, numfig=2, ver=0}
      mask prompts: PasoGrado2 "Tamaño de paso de grado"; numRBFs "Número de RBFs"; sigma2 "Sigma"; limitinf2 "Límite inferior"; limitsup2 "Límite superior"; numfig "Numero de figura"; ver "Visualización de gráfica VER=1"
  S3 : S-Function  FunctionName=fRBFgauss1optimal  Parameters=PasoGrado3,numRBFs,sigma3,limitinf3,limitsup3,numfig,ver  EnableBusSupport=off  mask{PasoGrado3=0.05, numRBFs=20, sigma3=(6-(-6))/(1.75*20), limitinf3=-6, limitsup3=6, numfig=2, ver=0}
      mask prompts: PasoGrado3 "Tamaño de paso de grado"; numRBFs "Número de RBFs"; sigma3 "Sigma"; limitinf3 "Límite inferior"; limitsup3 "Límite superior"; numfig "Numero de figura"; ver "Visualización de gráfica VER=1"
  MossyBlock1 : Outport
  MossyBlock2 : Outport  Port=2
  MossyBlock3 : Outport  Port=3
  MossyBlock4 : Outport  Port=4
  MossyBlock5 : Outport  Port=5
  MossyBlock6 : Outport  Port=6
  MossyBlock7 : Outport  Port=7
  wires:
  Demux/1 -> S1/1
  Demux/2 -> S2/1
  Demux/3 -> S3/1
  Demux/4 -> MossyBlock4/1
  Demux/6 -> MossyBlock6/1
  S1/1 -> MossyBlock1/1
  S2/1 -> MossyBlock2/1
  Demux/5 -> MossyBlock5/1
  Demux/7 -> MossyBlock7/1
  Posiciones  deseadas/1 -> MATLAB Fcn7/1
  MATLAB Fcn7/1 -> Demux/1
  S3/1 -> MossyBlock3/1
